simulink model "SimulinkAnalysisofCheetahTail"  (R2022a)
(part 9 of 21)

et239 = ITail.*t4476.*(t1368-t2524+t1430.*(t197-t537))+ITail.*t4522.*(t1396-t2573+t1430.*(t197-t537).*2.0)+ITail.*t4867.*(-t947+t1240.*(t105-t465)+t903.*(t534-t546))+ITail.*t4820.*(-t1017+(t1240.*(t105-t465))./2.0+(t903.*(t534-t546))./2.0);
et240 = -t5373-t5375+t6808+t6842+dth2.*(et236+et237+et238+et239);
et241 = dth1.*(t2206+t2293+t3526+t3530+t4005+t4009+t4143+t4171+t4449+t4451+t4529+t4532+t5099+t5136+t5370+t5402-t5421-t5435+t5502+t5509+t5733-t5771+t5975-t5985-t6076-t6167-t6233+t6255+t6314+t6319+t6434-t6681+t5394.*(t995+t1064-t1506+t1598-t1763-t1774)+t4672.*(-t2389+t3634+t1512.*(t105-t465).*9.53094055e-4)+t5304.*(t1332+t2368+t1512.*(t105-t465))+t6620.*(t1332+t2368+t1512.*(t105-t465))+ITail.*t4712.*(t1332+t2368+t1512.*(t105-t465))+ITail.*t4672.*(t1386+t2501+(t1512.*(t105-t465))./2.0));
et242 = -t5782.*(et223+et224)-dpsi1.*t6893+dth1.*t6895+dth2.*t6894-dx.*t6787+dy.*t6789-dz.*t6788+dphi2.*(dphi1.*(et225+et226+et227)+dth1.*(et228+et229)+dphi2.*(et230+et231)+dth2.*(et232+et233))-t5782.*(et234+et235)-t4883.*t6783-t5997.*t6472-t6472.*t6784;
et243 = -(-t2274+t4111+t1510.*(-t488+t603+dpsi1.*(t105-t465)+dth2.*(t103-t544))).*(t2271.*3.367829185e-3+t4083+t4096.*3.367829185e-3+t4196+t4213+t4606+t4623+t4689+t4691+t4696+t4698-t1505.*(-t488+t603+dpsi1.*(t105-t465)+dth2.*(t103-t544)).*3.367829185e-3);
et244 = -(t2271.*8.56645e-6+t4096.*8.56645e-6-t1505.*(-t488+t603+dpsi1.*(t105-t465)+dth2.*(t103-t544)).*8.56645e-6).*(-t2274+t4111+t1510.*(-t488+t603+dpsi1.*(t105-t465)+dth2.*(t103-t544)));
et245 = (-t3471+t4531+t4422.*(t105-t465)).*(t3448-t3523.*3.372786875e-3+t4196+t4213+t4309+t4326+t4528.*3.372786875e-3+t4689+t4691+t4696+t4698-t4415.*(t105-t465).*3.372786875e-3)+dphi1.*(et240+et241);
et246 = -(-t3471+t4531+t4422.*(t105-t465)).*(t3523.*9.53094055e-4-t4528.*9.53094055e-4+t4415.*(t105-t465).*9.53094055e-4);
et247 = -t4883.*(-t3614+t4341+t1510.*(-t488+t603+dpsi1.*(t105-t465)+dth2.*(t103-t544)).*8.56645e-6)-(t3523-t4528+t4415.*(t105-t465)).*(-t4087+t4644+t4422.*(t105-t465).*9.53094055e-4)+t6782.*(t3523-t4528+t4415.*(t105-t465))-Mb.*t5070.*(B_cg_H.*t1224+B_cg_H.*t1575+dphi2.*t1487+B_cg_H.*dth1.*t1047+B_cg_H.*dth2.*(t214-t541));
et248 = -ITail.*t4883.*(-t2361+t4138+(t1510.*(-t488+t603+dpsi1.*(t105-t465)+dth2.*(t103-t544)))./2.0)-Mt.*t5952.*(dphi1.*t2914+dphi2.*t3679+dpsi1.*t3774+dth1.*t2730+dth2.*(t451-t831+T_cg_H.*(t214-t541)))-ITail.*(-t3471+t4531+t4422.*(t105-t465)).*(t3523./2.0-t4528./2.0+(t4415.*(t105-t465))./2.0)+Mt.*t4796.*(-dphi1.*t1618+dphi2.*t2240+dth2.*t1495+dth1.*t2087)-ITail.*t5782.*(t3862./2.0+t3907./2.0-t4576./2.0-t4577./2.0+t4588./2.0+t4591./2.0)-ITail.*t5816.*t6472-Mt.*t5950.*(dphi1.*t2915+dphi2.*t3770+dpsi1.*t3780-dth2.*t2325-dth1.*t2763);
et249 = -Mb.*t5071.*(B_cg_H.*t1225+B_cg_H.*t1581+dphi2.*t1558-B_cg_H.*dth2.*t977-B_cg_H.*dth1.*t1037)-ITail.*(t3523-t4528+t4415.*(t105-t465)).*(-t3548+t4540+(t4422.*(t105-t465))./2.0)-ITail.*(t2271./2.0+t4096./2.0-(t1505.*(-t488+t603+dpsi1.*(t105-t465)+dth2.*(t103-t544)))./2.0).*(-t2274+t4111+t1510.*(-t488+t603+dpsi1.*(t105-t465)+dth2.*(t103-t544)))+Mb.*t4346.*(B_cg_H.*t629+B_cg_H.*t802+B_cg_H.*t902+dphi2.*t926);
et250 = t3499.*9.52624335e-4-t3772.*9.52624335e-4+t4352.*9.52624335e-4+t4542.*9.52624335e-4;
et251 = t1505.*(-t550+t693+t972-t1023+dpsi1.*(t214-t541)).*(-9.52624335e-4)-t4415.*(t197-t537).*9.52624335e-4;
et252 = t1917.*8.56645e-6-t2008.*8.56645e-6-t4105.*8.56645e-6+t977.*(-t488+t603+dpsi1.*(t105-t465)+dth2.*(t103-t544)).*8.56645e-6;
et253 = t1512.*(t553-t741+dpsi1.*(t103-t544)+dth2.*(t105-t465)).*8.56645e-6+t3113.*(t214-t541).*8.56645e-6;
et254 = -t1939+t2390+t2843-t2877+t3263+t3931+t4054+t4273+t4301-t4324+t4945+t4964+t5300-t5354-t5382+t5627+t5665+t5705-t5738+t5891+t6049-t6286+t6325+t6381-t6445-t6640+t6668-t6734+t4753.*(-t1129+t1139-t2082+t2110+t2123+t8.*t872.*(t534-t546))+t6106.*(-t1129+t1139-t2082+t2110+t2123+t8.*t872.*(t534-t546))+t4313.*(t2208+t2312-t3315+t3347+t3475+t1179.*(t103-t544).*8.56645e-6);
et255 = t4447.*(t2215-t2237+t3424+t3427-t3439+t8.*t872.*(t534-t546).*9.52624335e-4)+t4704.*(t1060+t1138-t1883+t1932+t2088+t1179.*(t103-t544))+t6105.*(t1060+t1138-t1883+t1932+t2088+t1179.*(t103-t544))+t4936.*(-t1262+t1701+t9.*t868.*(t105-t465));
et256 = t4447.*(t1645+t1965+t2072+t2220-t2242-t2409-t2483-t2504-t3093+t3155+t3261+t3432+t3437-t3442+t1179.*(t103-t544).*3.36554e-3+t3.*t575.*(t105-t465).*3.36554e-3+t8.*t872.*(t534-t546).*3.372816795e-3);
et257 = t4454.*(-t2388+t3008+t9.*t868.*(t105-t465).*9.53094055e-4);
et258 = t4313.*(t1645+t2037-t2064+t2156+t2227-t2409-t2483-t2504-t3244+t3270-t3276+t3299+t3312+t3413+t1179.*(t103-t544).*3.367829185e-3+t3.*t575.*(t105-t465).*3.36554e-3+t8.*t872.*(t534-t546).*3.36554e-3)+t6616.*(-t1331+t2317+t1510.*(t103-t544));
et259 = (-t1331+t2317+t1510.*(t103-t544)).*(-t2218+t2342+t3054+t3096+t3121+t3131)+Mt.*(t433-t828+T_cg_H.*(t197-t537)).*(-t130+t436+t523-t657+t769)+ITail.*t4459.*(-t1129+t1139-t2082+t2110+t2123+t8.*t872.*(t534-t546))+ITail.*t4447.*(-t1189+t1195-t2210+t2241+t2248+(t8.*t872.*(t534-t546))./2.0)+ITail.*t4350.*(t1060+t1138-t1883+t1932+t2088+t1179.*(t103-t544))+ITail.*t4313.*(t1143+t1194-t1959+t2038+t2175+(t1179.*(t103-t544))./2.0)+ITail.*t4490.*(-t1262+t1701+t9.*t868.*(t105-t465))+ITail.*t4454.*(-t1355+t1789+(t9.*t868.*(t105-t465))./2.0)+B_cg_H.*Mb.*t11.*t641.*t2563;
et260 = t1304.*-2.0+t1746.*2.0-t3331.*2.0+t4025.*2.0-t6090.*(t1250-t1261+t1761-t2083-t2111+t1037.*(t103-t544)).*2.0+t4737.*t4834.*2.0+t4408.*t5597.*2.0-t3961.*t6604.*2.0-t4834.*t6091.*2.0+t4408.*t6608.*2.0+t4551.*(-t1018+t1426+t1431-t1446+t3.*t496.*(t105-t465)).*2.0+t6089.*(-t1018+t1426+t1431-t1446+t3.*t496.*(t105-t465)).*2.0-(-t2621+t3659+t1510.*(t103-t544).*8.56645e-6).*(t1250-t1261+t1761-t2083-t2111+t1037.*(t103-t544)).*2.0;
et261 = t3961.*(-t2058+t2688+t2700-t2718+t3.*t496.*(t105-t465).*9.53094055e-4).*2.0-t6607.*(-t1331+t2317+t1510.*(t103-t544)).*2.0+(-t1331+t2317+t1510.*(t103-t544)).*(t2514-t2518+t3160+t3266+t3501+t3510).*2.0-ITail.*(-t1412+t2419+(t1510.*(t103-t544))./2.0).*(t1250-t1261+t1761-t2083-t2111+t1037.*(t103-t544)).*2.0-ITail.*(-t1331+t2317+t1510.*(t103-t544)).*(t1334-t1354+t1851-t2212-t2243+(t1037.*(t103-t544))./2.0).*2.0;
et262 = Mt.*t1734.*(t433-t828+T_cg_H.*(t197-t537)).*2.0+ITail.*t4452.*t4834.*2.0+ITail.*t4408.*t4900.*2.0+ITail.*t4071.*(-t1018+t1426+t1431-t1446+t3.*t496.*(t105-t465)).*2.0+ITail.*t3961.*(-t993+t1535+t1540-t1552+(t3.*t496.*(t105-t465))./2.0).*2.0+Mb.*t15.*t721.*(t197-t537).*2.0;
et263 = t983.*2.0-t1624.*2.0+t2420.*2.0-t3841.*2.0-t4737.*(-t1129+t1139-t2082+t2110+t2123+t8.*t872.*(t534-t546)).*2.0+t6091.*(-t1129+t1139-t2082+t2110+t2123+t8.*t872.*(t534-t546)).*2.0-t3961.*t4936.*2.0-t4454.*t4551.*2.0-t4454.*t6089.*2.0-t4408.*(t2215-t2237+t3424+t3427-t3439+t8.*t872.*(t534-t546).*9.52624335e-4).*2.0+t6090.*(t1060+t1138-t1883+t1932+t2088+t1179.*(t103-t544)).*2.0;
et264 = t3961.*(t1799+t1965+t2037-t2064+t2072-t2613-t2696-t2723-t3093+t3155+t3261+t3270-t3276+t3312+t1179.*(t103-t544).*3.36554e-3+t3.*t575.*(t105-t465).*3.372786875e-3+t8.*t872.*(t534-t546).*3.36554e-3).*2.0;
et265 = (-t1331+t2317+t1510.*(t103-t544)).*(t1645+t2037-t2064+t2156+t2227-t2409-t2483-t2504-t3244+t3270-t3276+t3299+t3312+t3413+t1179.*(t103-t544).*3.367829185e-3+t3.*t575.*(t105-t465).*3.36554e-3+t8.*t872.*(t534-t546).*3.36554e-3).*2.0;
et266 = t4408.*(t1645+t1965+t2072+t2220-t2242-t2409-t2483-t2504-t3093+t3155+t3261+t3432+t3437-t3442+t1179.*(t103-t544).*3.36554e-3+t3.*t575.*(t105-t465).*3.36554e-3+t8.*t872.*(t534-t546).*3.372816795e-3).*-2.0;
et267 = (-t2621+t3659+t1510.*(t103-t544).*8.56645e-6).*(t1060+t1138-t1883+t1932+t2088+t1179.*(t103-t544)).*2.0+(-t1331+t2317+t1510.*(t103-t544)).*(t2208+t2312-t3315+t3347+t3475+t1179.*(t103-t544).*8.56645e-6).*2.0+Mt.*t1528.*(t433-t828+T_cg_H.*(t197-t537)).*2.0+ITail.*(-t1412+t2419+(t1510.*(t103-t544))./2.0).*(t1060+t1138-t1883+t1932+t2088+t1179.*(t103-t544)).*2.0;
et268 = ITail.*(-t1331+t2317+t1510.*(t103-t544)).*(t1143+t1194-t1959+t2038+t2175+(t1179.*(t103-t544))./2.0).*2.0-ITail.*t4452.*(-t1129+t1139-t2082+t2110+t2123+t8.*t872.*(t534-t546)).*2.0-ITail.*t4408.*(-t1189+t1195-t2210+t2241+t2248+(t8.*t872.*(t534-t546))./2.0).*2.0-ITail.*t3961.*t4490.*2.0-ITail.*t4071.*t4454.*2.0+Mb.*t11.*t15.*t542.*(t197-t537).*2.0;
et269 = t3961.*(t2059-t2952+t3009+t3.*t818.*(t105-t465).*9.53094055e-4+t3.*t872.*(t103-t544).*9.53094055e-4).*2.0+t4737.*t4849.*2.0+t4408.*t5607.*2.0-t3961.*t6614.*2.0-t4849.*t6091.*2.0+t4408.*t6619.*2.0;
et270 = (-t1331+t2317+t1510.*(t103-t544)).*(t2202+t2564+t3719+t817.*(t214-t541).*8.56645e-6+t977.*(t103-t544).*8.56645e-6+t1512.*(t105-t465).*8.56645e-6).*-2.0;
et271 = (-t2621+t3659+t1510.*(t103-t544).*8.56645e-6).*(t1053+t1332+t2368+t817.*(t214-t541)+t977.*(t103-t544)+t1512.*(t105-t465)).*-2.0+t4551.*(t1019-t1651+t1702+t3.*t818.*(t105-t465)+t3.*t872.*(t103-t544)).*2.0+t6089.*(t1019-t1651+t1702+t3.*t818.*(t105-t465)+t3.*t872.*(t103-t544)).*2.0-t6618.*(-t1331+t2317+t1510.*(t103-t544)).*2.0-t6090.*(t1053+t1332+t2368+t817.*(t214-t541)+t977.*(t103-t544)+t1512.*(t105-t465)).*2.0;
et272 = ITail.*t4071.*(t1019-t1651+t1702+t3.*t818.*(t105-t465)+t3.*t872.*(t103-t544)).*2.0+ITail.*t3961.*(t994-t1742+t1790+(t3.*t818.*(t105-t465))./2.0+(t3.*t872.*(t103-t544))./2.0).*2.0+Mt.*t2174.*(t433-t828+T_cg_H.*(t197-t537)).*2.0+ITail.*t4452.*t4849.*2.0+ITail.*t4408.*t4908.*2.0+Mt.*t1531.*t1619.*2.0+Mt.*t2319.*(t431+t909+T_cg_H.*(t195-t634)).*2.0-ITail.*(-t1412+t2419+(t1510.*(t103-t544))./2.0).*(t1053+t1332+t2368+t817.*(t214-t541)+t977.*(t103-t544)+t1512.*(t105-t465)).*2.0;
et273 = ITail.*(-t1331+t2317+t1510.*(t103-t544)).*(t1141+t1386+t2501+(t817.*(t214-t541))./2.0+(t977.*(t103-t544))./2.0+(t1512.*(t105-t465))./2.0).*-2.0+Mb.*t15.*t485.*t557.*2.0+Mb.*t15.*t925.*(t197-t537).*2.0+Mb.*t15.*t964.*(t195-t634).*2.0;
et274 = t1242.*2.0+t1977.*2.0+t1979.*2.0+t3248.*2.0+t4141.*2.0+t4160.*2.0+t3961.*(t1667-t2347+t2438+t2447+t3012+t3022+t3458+t3543+t3587+t3594+t3600+t3621).*2.0-t4408.*(t1568-t2347+t2657+t2663+t2871+t2875+t3458+t3621+t3638+t3697+t3735+t3745).*2.0+(-t1331+t2317+t1510.*(t103-t544)).*(t1568-t2404-t2412+t2528+t2871+t2875+t3543+t3550+t3587+t3594+t3600+t3746).*2.0+t3961.*t4549.*2.0+t3967.*t4551.*2.0+t4737.*t4972.*2.0+t3967.*t6089.*2.0-t4382.*t6090.*2.0-t4972.*t6091.*2.0+t4408.*(t2590+t2616-t3627+t3698+t3738+t3764).*2.0-t4382.*(-t2621+t3659+t1510.*(t103-t544).*8.56645e-6).*2.0;
et275 = t4736.*(-t1331+t2317+t1510.*(t103-t544)).*-2.0-ITail.*t4416.*(-t1331+t2317+t1510.*(t103-t544)).*2.0-ITail.*t4382.*(-t1412+t2419+(t1510.*(t103-t544))./2.0).*2.0+ITail.*t3961.*t4072.*2.0+ITail.*t3967.*t4071.*2.0+ITail.*t4408.*t5013.*2.0+ITail.*t4452.*t4972.*2.0;
et276 = t1917.*3.367829185e-3-t2008.*3.367829185e-3-t3815+t4042-t4074-t4105.*3.367829185e-3+t4135-t4403+t4404-t4462+t4605-t4647+t1505.*(-t550+t693+t972-t1023+dpsi1.*(t214-t541)).*3.36554e-3;
et277 = t977.*(-t488+t603+dpsi1.*(t105-t465)+dth2.*(t103-t544)).*3.367829185e-3+t1512.*(t553-t741+dpsi1.*(t103-t544)+dth2.*(t105-t465)).*3.367829185e-3+t3113.*(t214-t541).*3.367829185e-3;
et278 = t4435.*(t103-t544).*3.36554e-3+t4415.*(t197-t537).*3.36554e-3;
et279 = -t1703+t2015+t3449-t3787+t3916+t3923+t3947-t4371-t4401+t4469+t4493+t5371+t5372+t5404+t5405+t5748+t5749+t5781+t5808+t5986+t5988+t5989+t6103-t6433-t6448-t6645+t6646+t6776+t6779+t6090.*(t867+t1059-t1646-t1705+t1938-t2002)+t4787.*(-t1129+t1139-t2082+t2110+t2123+t8.*t872.*(t534-t546));
et280 = t4454.*(t1970-t1971+t2487+t3161-t3236-t3794-t3817+t1240.*(t105-t465).*3.372786875e-3+t903.*(t534-t546).*3.372786875e-3)+t4551.*(t753+t991-t1771-t1957+t1181.*(t105-t465)+t11.*t381.*(t534-t546))+t6089.*(t753+t991-t1771-t1957+t1181.*(t105-t465)+t11.*t381.*(t534-t546));
et281 = t4476.*(t2215-t2237+t3424+t3427-t3439+t8.*t872.*(t534-t546).*9.52624335e-4)+t6091.*(t1176-t1366+t2434+t2435-t2899+t1430.*(t539+t641));
et282 = t4476.*(t1645+t1965+t2072+t2220-t2242-t2409-t2483-t2504-t3093+t3155+t3261+t3432+t3437-t3442+t1179.*(t103-t544).*3.36554e-3+t3.*t575.*(t105-t465).*3.36554e-3+t8.*t872.*(t534-t546).*3.372816795e-3);
et283 = t4454.*(-t1974+t1240.*(t105-t465).*9.53094055e-4+t903.*(t534-t546).*9.53094055e-4);
et284 = t3961.*(t1786+t1810+t1964+t2047+t2152-t2401-t2797-t2860-t3076+t3167-t3232-t3278+t3582+t3583-t3837+t1430.*(t539+t641).*3.36554e-3+t1181.*(t105-t465).*3.372786875e-3+t11.*t381.*(t534-t546).*3.372786875e-3);
et285 = t3961.*(t1784+t2057-t3080-t3287+t1181.*(t105-t465).*9.53094055e-4+t11.*t381.*(t534-t546).*9.53094055e-4)+t4936.*(-t947+t1240.*(t105-t465)+t903.*(t534-t546))+ITail.*t4490.*(-t947+t1240.*(t105-t465)+t903.*(t534-t546))+ITail.*t4454.*(-t1017+(t1240.*(t105-t465))./2.0+(t903.*(t534-t546))./2.0);
et286 = ITail.*t4522.*(-t1129+t1139-t2082+t2110+t2123+t8.*t872.*(t534-t546))+ITail.*t4476.*(-t1189+t1195-t2210+t2241+t2248+(t8.*t872.*(t534-t546))./2.0)+ITail.*t4071.*(t753+t991-t1771-t1957+t1181.*(t105-t465)+t11.*t381.*(t534-t546))+ITail.*t3961.*(t865+t1086-t1855-t2076+(t1181.*(t105-t465))./2.0+(t11.*t381.*(t534-t546))./2.0)+B_cg_H.*Mb.*t11.*t641.*t3206;
et287 = t2824.*9.53094055e-4+t3522.*9.53094055e-4+t4272.*9.53094055e-4+t4281.*9.53094055e-4-t4519.*9.53094055e-4;
et288 = t4435.*(t103-t544).*(-9.53094055e-4);
et289 = t2824.*3.372786875e-3+t3178+t3247+t3522.*3.372786875e-3+t4061+t4145+t4223+t4231+t4272.*3.372786875e-3+t4281.*3.372786875e-3+t4318+t4342+t4462+t4487;
et290 = t4519.*(-3.372786875e-3)+t4626+t4647-t4435.*(t103-t544).*3.372786875e-3;
et291 = t3178+t3247+t3499.*3.372816795e-3-t3772.*3.372816795e-3+t3815+t4074+t4223+t4231+t4318+t4342+t4352.*3.372816795e-3+t4403+t4407+t4542.*3.372816795e-3+t4609+t4639;
et292 = t1505.*(-t550+t693+t972-t1023+dpsi1.*(t214-t541)).*(-3.372816795e-3)-t4415.*(t197-t537).*3.372816795e-3;
et293 = t5782.*(et250+et251)-(-t2274+t4111+t1510.*(-t488+t603+dpsi1.*(t105-t465)+dth2.*(t103-t544))).*(et252+et253)+dy.*(t4877-t5660-t5824+dphi2.*(t843-t1421+t1685-t2937+Mt.*t420.*(t451-t831+T_cg_H.*(t214-t541))+B_cg_H.*Mb.*t420.*(t214-t541)))-t6217.*(-t4087+t4644+t4422.*(t105-t465).*9.53094055e-4)+dphi2.*t6894+dpsi1.*t6897-dx.*t6569+t6217.*t6782;
et294 = -dth1.*(t4786-t4790+t6845-t6880-t6885+dphi1.*(et254+et255+et256+et257+et258+et259)+dx.*(-t754+t1167-t1635+t2574+Mt.*t9.*t10.*(t433-t828+T_cg_H.*(t197-t537))+B_cg_H.*Mb.*t9.*t10.*(t197-t537)))-dz.*(t4851-t5727+t5821+dth2.*(t886-t1360+t1759-t2791+Mt.*t421.*(t431+t909+T_cg_H.*(t195-t634))+B_cg_H.*Mb.*t421.*(t195-t634)))-t6783.*(t1917-t2008-t4105+t977.*(-t488+t603+dpsi1.*(t105-t465)+dth2.*(t103-t544))+t1512.*(t553-t741+dpsi1.*(t103-t544)+dth2.*(t105-t465))+t3113.*(t214-t541));
et295 = -t5997.*(t3419+t3772-t4352-t4542+t1505.*(-t550+t693+t972-t1023+dpsi1.*(t214-t541))+t4415.*(t197-t537))-t6784.*(t3419+t3772-t4352-t4542+t1505.*(-t550+t693+t972-t1023+dpsi1.*(t214-t541))+t4415.*(t197-t537))-dth2.*(dth1.*(et260+et261+et262)+dphi1.*(et263+et264+et265+et266+et267+et268)+dth2.*(et269+et270+et271+et272+et273)+dphi2.*(et274+et275))-(-t2274+t4111+t1510.*(-t488+t603+dpsi1.*(t105-t465)+dth2.*(t103-t544))).*(et276+et277+et278);
et296 = -dphi1.*(t4850-t6848-t6876-t6878+dphi1.*(et279+et280+et281+et282+et283+et284+et285+et286)+dz.*(t838-t1413+t1672-t2921+Mt.*t420.*(t433-t828+T_cg_H.*(t197-t537))+B_cg_H.*Mb.*t420.*(t197-t537)));
et297 = -(-t3614+t4341+t1510.*(-t488+t603+dpsi1.*(t105-t465)+dth2.*(t103-t544)).*8.56645e-6).*(t1917-t2008-t4105+t977.*(-t488+t603+dpsi1.*(t105-t465)+dth2.*(t103-t544))+t1512.*(t553-t741+dpsi1.*(t103-t544)+dth2.*(t105-t465))+t3113.*(t214-t541))-(-t3471+t4531+t4422.*(t105-t465)).*(et287+et288)-(-t3471+t4531+t4422.*(t105-t465)).*(et289+et290)+t5782.*(et291+et292);
et298 = -Mt.*t5952.*(dphi1.*t1528-dpsi1.*t2319+dth1.*t1734+dth2.*t2174+dphi2.*(t451-t831+T_cg_H.*(t214-t541)))-ITail.*(-t2361+t4138+(t1510.*(-t488+t603+dpsi1.*(t105-t465)+dth2.*(t103-t544)))./2.0).*(t1917-t2008-t4105+t977.*(-t488+t603+dpsi1.*(t105-t465)+dth2.*(t103-t544))+t1512.*(t553-t741+dpsi1.*(t103-t544)+dth2.*(t105-t465))+t3113.*(t214-t541))+Mb.*t4346.*(B_cg_H.*t259+B_cg_H.*t628+B_cg_H.*t806+B_cg_H.*dth2.*t557)-ITail.*t6217.*(-t3548+t4540+(t4422.*(t105-t465))./2.0);
et299 = Mt.*t5950.*(-dphi1.*t1381+dphi2.*t2325+dth1.*t1727+dth2.*(t431+t909+T_cg_H.*(t195-t634))+dpsi1.*(t433-t828+T_cg_H.*(t197-t537)))+Mt.*t4796.*(dphi1.*t876+dphi2.*t1495-dth1.*t1620+dth2.*t1619)+ITail.*t5782.*(t3499./2.0-t3772./2.0+t4352./2.0+t4542./2.0-(t1505.*(-t550+t693+t972-t1023+dpsi1.*(t214-t541)))./2.0-(t4415.*(t197-t537))./2.0);
et300 = -ITail.*(-t2274+t4111+t1510.*(-t488+t603+dpsi1.*(t105-t465)+dth2.*(t103-t544))).*(t1917./2.0-t2008./2.0-t4105./2.0+(t977.*(-t488+t603+dpsi1.*(t105-t465)+dth2.*(t103-t544)))./2.0+(t1512.*(t553-t741+dpsi1.*(t103-t544)+dth2.*(t105-t465)))./2.0+(t3113.*(t214-t541))./2.0)-ITail.*t5816.*(t3419+t3772-t4352-t4542+t1505.*(-t550+t693+t972-t1023+dpsi1.*(t214-t541))+t4415.*(t197-t537))-Mb.*t5070.*(B_cg_H.*t731+B_cg_H.*t1099+B_cg_H.*t1113+B_cg_H.*dth1.*t721+B_cg_H.*dth2.*t925);
et301 = -ITail.*(-t3471+t4531+t4422.*(t105-t465)).*(t2824./2.0+t3522./2.0+t4272./2.0+t4281./2.0-t4519./2.0-(t4435.*(t103-t544))./2.0)+Mb.*t5071.*(B_cg_H.*t732+B_cg_H.*t1029+B_cg_H.*t1102+B_cg_H.*dth1.*t675+B_cg_H.*dth2.*(t195-t634));
mt1 = [-dphi2.*t6787-dphi1.*t6791+dpsi1.*t6790-dth2.*t6569-dth1.*t6792-dz.*t4995-dy.*(t4189-t4598)+Mb.*t377.*t5071+Mb.*t415.*t5070+Mm.*t377.*t4274-Mm.*t415.*t4276+Mt.*t377.*t5950+Mt.*t415.*t5952-dth1.*dx.*(t48.*-2.0-t49.*2.0-t50.*2.0+t284.*2.0+t287.*2.0+t288.*2.0+t290.*2.0+t293.*2.0+t294.*2.0)-Mb.*dth1.*t5.*t4346-Mm.*dth1.*t5.*t2062-Mt.*dth1.*t5.*t4796];
mt2 = [dz.*(t4752-dphi1.*(t4078-t4081))+dth2.*(t4877-t5660-t5824+dphi2.*(t843-t1421+t1685-t2937+Mt.*t420.*(t451-t831+T_cg_H.*(t214-t541))+B_cg_H.*Mb.*t420.*(t214-t541)))-dy.*(t4512+dth1.*(t289.*2.0+t291.*2.0+t292.*2.0-t665.*2.0-t667.*2.0-t669.*2.0+t795.*2.0+t797.*2.0+t799.*2.0))+dphi2.*t6789+dphi1.*t6795+dpsi1.*t6793-dth1.*t6797-dx.*(t4189-t4598)+Mb.*t414.*t4346+Mb.*t1205.*t5070-Mb.*t1389.*t5071+Mm.*t414.*t2062-Mm.*t1205.*t4276-Mm.*t1389.*t4274+Mt.*t414.*t4796+Mt.*t1205.*t5952-Mt.*t1389.*t5950];
mt3 = [dy.*(t4752-dphi1.*(t4078-t4081))+dz.*(t4512-dth1.*(t283.*2.0+t285.*2.0+t286.*2.0-t664.*2.0-t666.*2.0-t668.*2.0+t772.*2.0+t774.*2.0+t776.*2.0))-dphi2.*t6788+dphi1.*t6796-dpsi1.*t6794-dth1.*t6798-dx.*t4995-dth2.*(t4851-t5727+t5821+dth2.*(t886-t1360+t1759-t2791+Mt.*t421.*(t431+t909+T_cg_H.*(t195-t634))+B_cg_H.*Mb.*t421.*(t195-t634)))+Mb.*t376.*t4346-Mb.*t1265.*t5071-Mb.*t1388.*t5070+Mm.*t376.*t2062-Mm.*t1265.*t4274+Mm.*t1388.*t4276+Mt.*t376.*t4796-Mt.*t1265.*t5950-Mt.*t1388.*t5952;et159+et160+et161+et162+et163+et164+et165+et166+et167;et199+et200+et201+et202+et203+et204+et205];
mt4 = [-dphi2.*t6893-dphi1.*t6898+dth2.*t6897-dth1.*t6899+dx.*t6790+dy.*t6793-dz.*t6794+dpsi1.*(dx.*(Mb.*t5.*t9.*t3836.*2.0+Mb.*t4.*t5.*t3848.*2.0+Mm.*t4.*t5.*t1394.*2.0-Mm.*t5.*t9.*t1470.*2.0+Mt.*t5.*t9.*t4344.*2.0+Mt.*t4.*t5.*t4357.*2.0)-dth1.*(et206+et207+et208)+dy.*(Mb.*t381.*t3848.*2.0-Mb.*t420.*t3836.*2.0+Mm.*t381.*t1394.*2.0+Mm.*t420.*t1470.*2.0+Mt.*t381.*t4357.*2.0-Mt.*t420.*t4344.*2.0)+dz.*(Mb.*t382.*t3836.*-2.0+Mb.*t421.*t3848.*2.0+Mm.*t421.*t1394.*2.0+Mm.*t382.*t1470.*2.0-Mt.*t382.*t4344.*2.0+Mt.*t421.*t4357.*2.0)+dth2.*(et215+et216+et217+et218)-dphi2.*(et219+et220)+dphi1.*(et221+et222));et242+et243+et244+et245+et246+et247+et248+et249;et293+et294+et295+et296+et297+et298+et299+et300+et301];
C = [mt1;mt2;mt3;mt4];
end
